simulink model "dlbpid"  (Simulink 8.3)
settings: Solver=ode45  StartTime=0.0  StopTime=10.0  RelTol=1e-3
settings Model: Creator=Administrator  LastModifiedBy=Administrator
settings OptimizationCC: ExpressionDepthLimit=2147483647
settings DebuggingCC: FcnCallInpInsideContextMsg=EnableAllAsWarning

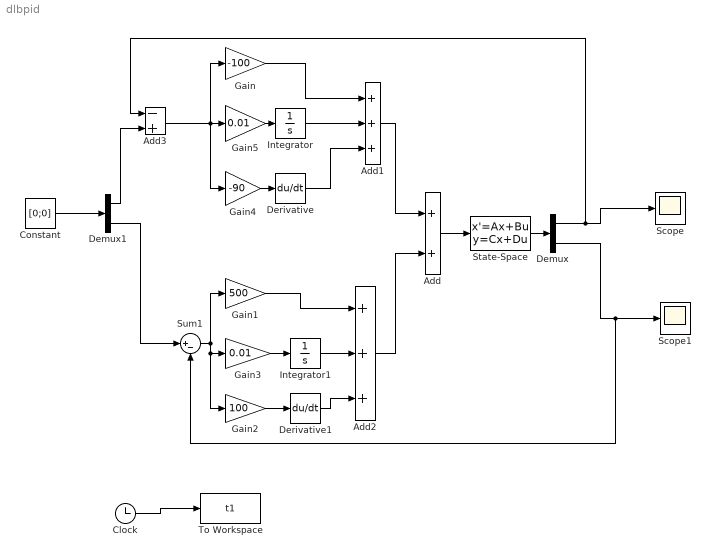
== system dlbpid ==
  Add : Sum
  Add1 : Sum  Inputs=+++
  Add2 : Sum  Inputs=+++
  Add3 : Sum  Inputs=-+
  Clock : Clock
  Constant : Constant  Value=[0;0]
  Demux : Demux  Outputs=2
  Demux1 : Demux  Outputs=2
  Derivative : Derivative
  Derivative1 : Derivative
  Gain : Gain  Gain=-100
  Gain1 : Gain  Gain=500
  Gain2 : Gain  Gain=100
  Gain3 : Gain  Gain=0.01
  Gain4 : Gain  Gain=-90
  Gain5 : Gain  Gain=0.01
  Integrator : Integrator
  Integrator1 : Integrator
  Scope : Scope
      settings: SaveName=location
  Scope1 : Scope
      settings: SaveName=angle
  State-Space : StateSpace  A=[0 1 0 0;0 0 0.717 0;0 0 0 1;0 0 15.777 0]  B=[0;0.975;0;1.464]  C=[1 0 0 0;0 0 1 0]  D=[0;0]  X0=[0;0;0.1;0]
  Sum1 : Sum  Inputs=|+-
  To Workspace : ToWorkspace  VariableName=t1  SampleTime=-1
  wires:
  Demux1/2 -> Sum1/1
  Sum1/1 -> Gain2/1, Gain3/1, Gain1/1
  Gain2/1 -> Derivative1/1
  Gain3/1 -> Integrator1/1
  Gain1/1 -> Add2/1
  Demux1/1 -> Add3/2
  Add3/1 -> Gain5/1, Gain/1, Gain4/1
  Gain4/1 -> Derivative/1
  Gain5/1 -> Integrator/1
  Gain/1 -> Add1/1
  Add1/1 -> Add/1
  Add2/1 -> Add/2
  Add/1 -> State-Space/1
  State-Space/1 -> Demux/1
  Demux/1 -> Add3/1, Scope/1
  Demux/2 -> Sum1/2, Scope1/1
  Constant/1 -> Demux1/1
  Integrator/1 -> Add1/2
  Derivative/1 -> Add1/3
  Integrator1/1 -> Add2/2
  Derivative1/1 -> Add2/3
  Clock/1 -> To Workspace/1
